simulink model "BMS_CL_Harness_advancedcell"  (R2015b)
settings: Solver=FixedStepDiscrete  StartTime=0.0  StopTime=final_time  FixedStep=BMSk_stepSize  RelTol=1e-3
values from neighbouring files (symbols this model uses):
  charge_cycle = 3    [BMS_test_cases.m]
undefined symbols (not defined in the file or in its folder): BMSc_airTemperature, BMSc_cabinTemperature, BMSk_stepSize, cell_ocvs_sampling, cell_socs_sampling, cell_temps_sampling, cell_voltages_sampling, inital_outlet_temperature, initial_cell_ocvs, initial_cell_socs, initial_cell_temps, initial_cell_voltages, initial_pack_current, initial_pack_soc, initial_pack_voltage, initial_vehicle_side_voltage, pack_current_sampling, pack_soc_sampling, pack_voltage_sampling, sigbuilder_block, vehicle_side_voltage_sampling
libraries: simulink x3
(part 1 of 2)
settings Model: PauseTimes=22  Creator=ms2zwt  LastModifiedBy=nctzv8
settings ConfigSet: Description=OpenECU configuration set for code generation under RTW-EC.
settings SolverCC: PositivePriorityOrder=on
settings DataIOCC: SaveFormat=Array  SignalLoggingSaveFormat=ModelDataLogs  SignalLogging=off
settings OptimizationCC: DefaultParameterBehavior=Inlined  InlineInvariantSignals=on  ExpressionDepthLimit=2147483647  StateBitsets=on  DataBitsets=on  ZeroExternalMemoryAtStartup=off  ZeroInternalMemoryAtStartup=off  NoFixptDivByZeroProtection=on  EfficientFloat2IntCast=on  OptimizeModelRefInitCode=on  LifeSpan=1
settings DebuggingCC: SaveWithParameterizedLinksMsg=none  UnderspecifiedInitializationDetection=Classic  MergeDetectMultiDrivingBlocksExec=none  SignalResolutionControl=TryResolveAllWithWarning  MultiTaskDSMMsg=warning  MultiTaskCondExecSysMsg=none  SingleTaskRateTransMsg=error  CheckMatrixSingularityMsg=warning  VectorMatrixConversionMsg=warning  FcnCallInpInsideContextMsg=UseLocalSettings  SignalLabelMismatchMsg=warning  StateNameClashWarn=warning
settings HardwareCC: ProdBitPerPointer=32  ProdLargestAtomicInteger=Long  ProdLargestAtomicFloat=Double  ProdEndianess=BigEndian  ProdWordSize=32  ProdHWDeviceType=Freescale->32-bit PowerPC  TargetIntDivRoundTo=Zero  TargetEndianess=BigEndian  TargetHWDeviceType=Freescale->32-bit PowerPC  ProdEqTarget=off
settings RTWCC: SystemTargetFile=openecu_ert.tlc  MakeCommand=make_rtw optimized_floating_point=1  TemplateMakefile=openecu_ert_r2015b_64.tmf  Description=OpenECU Platform Target (ERT, optimised floating-point code)  RetainRTWFile=on  IncludeHyperlinkInReport=on
settings CodeAppCC: ForceParamTrailComments=on  IgnoreCustomStorageClasses=off  SimulinkDataObjDesc=on  CustomSymbolStrType=$N$R$M  InsertBlockDesc=on  InternalIdentifier=Classic
settings STFCustomTargetCC: TargetLibSuffix=.a  GenerateSampleERTMain=on  ConcurrentExecutionCompliant=off  IncludeMdlTerminateFcn=off  GeneratePreprocessorConditionals=Use local settings  CombineOutputUpdateFcns=on  IncludeFileDelimiter=UseQuote  ERTCustomFileBanners=on  SupportContinuousTime=off  MATLABClassNameForMDSCustomization=Simulink.SoftwareTarget.ERTCustomization  CPPClassGenCompliant=off  GRTInterface=off  SystemTargetFile=openecu_ert.tlc
settings ERTTargetCC: GenerateSampleERTMain=on  ParMdlRefBuildCompliant=off  CompOptLevelCompliant=off  ConcurrentExecutionCompliant=off  IncludeMdlTerminateFcn=off  ERTFirstTimeCompliant=off  IncludeFileDelimiter=UseQuote  SupportNonInlinedSFcns=on  ModelStepFunctionPrototypeControlCompliant=off  CPPClassGenCompliant=off  UseToolchainInfoCompliant=off  ExtModeMexFile=noextcomm  InlinedParameterPlacement=NonHierarchical  ERTSrcFileBannerTemplate=oe_code_c_template.cgt  ERTHdrFileBannerTemplate=oe_code_h_template.cgt  ERTDataSrcFileTemplate=oe_data_c_template.cgt  ERTDataHdrFileTemplate=oe_data_h_template.cgt  ERTCustomFileTemplate=example_file_process.tlc  GlobalDataDefinition=InSeparateSourceFile  GlobalDataReference=InSeparateHeaderFile  EnableUserReplacementTypes=on

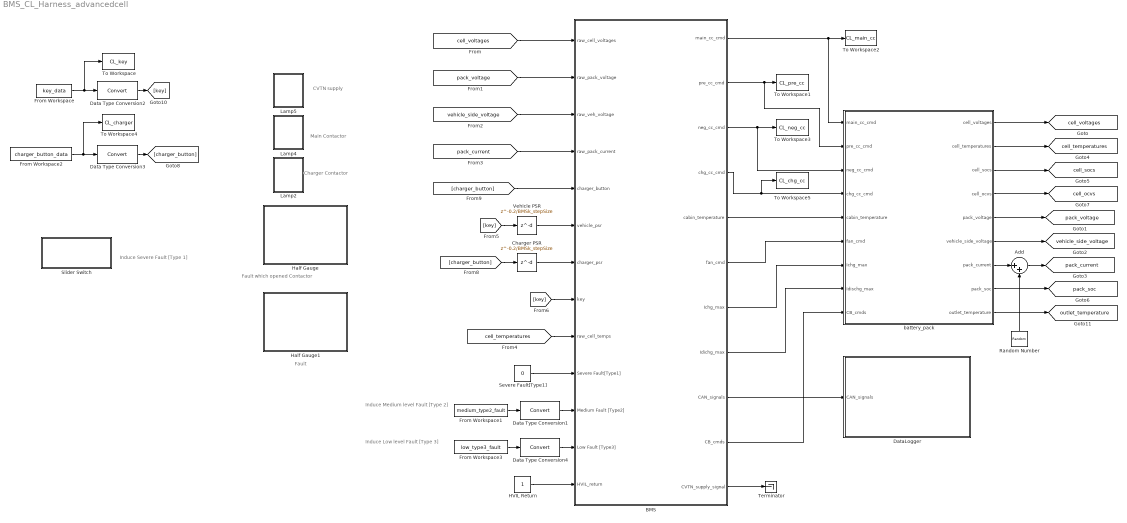
== system BMS_CL_Harness_advancedcell ==
  note: Fault
  note: Induce Medium level Fault
      | [Type 2]
  note: Induce Severe Fault
      | [Type 1]
  note: CVTN supply
  note: Charger Contactor
  note: Main Contactor
  note: Fault which opened Contactor
  note: Induce Low level Fault
      | [Type 3]
  Add : Sum  Inputs=|++
  BMS : Subsystem
  Charger PSR : Delay  DelayLength=0.2/BMSk_stepSize
  Data Type Conversion{1..4} (4 alike) : DataTypeConversion
  DataLogger : Subsystem
  From Workspace : FromWorkspace  VariableName=key_data  SampleTime=BMSk_stepSize
  From Workspace1 : FromWorkspace  VariableName=medium_type2_fault  SampleTime=BMSk_stepSize
  From Workspace2 : FromWorkspace  VariableName=charger_button_data  SampleTime=BMSk_stepSize
  From Workspace3 : FromWorkspace  VariableName=low_type3_fault  SampleTime=BMSk_stepSize
  HVIL Return : Constant  OutDataTypeStr=double  SampleTime=-1
  Half Gauge : Subsystem  DialogController=hmiCreateDDGDialog  IsWebBlock=on  mask(MWDashboardBlock){webBlockId=389, webBlockType=semicirculargauge, ShowInLibBrowser=on, ShowInitialText=on, HMISrcModelName=BMS_CL_Harness_advancedcell}
      mask prompts: webBlockId "WebBlock Id"; webBlockType "WebBlock Type"; HMISrcModelName "Source Model"
      mask Help: helpview([docroot '/mapfiles/simulink.map'], 'hmi_half_gauge')
      mask Display:
      | if strcmp(get_param(bdroot(gcb),'BlockDiagramType'), 'library')
      |     image([(matlabroot) '/toolbox/simulink/hmi/icons/SemicircularGauge.png']);
      | end
  Half Gauge1 : Subsystem  DialogController=hmiCreateDDGDialog  IsWebBlock=on  mask(MWDashboardBlock){webBlockId=61f53593-50c6-4eb0-9ab9-b848c630297d, webBlockType=semicirculargauge, ShowInLibBrowser=on, ShowInitialText=on, HMISrcModelName=BMS_CL_Harness_advancedcell}
      mask prompts: webBlockId "WebBlock Id"; webBlockType "WebBlock Type"; HMISrcModelName "Source Model"
      mask Help: helpview([docroot '/mapfiles/simulink.map'], 'hmi_half_gauge')
      mask Display:
      | if strcmp(get_param(bdroot(gcb),'BlockDiagramType'), 'library')
      |     image([(matlabroot) '/toolbox/simulink/hmi/icons/SemicircularGauge.png']);
      | end
  Lamp2 : Subsystem  DialogController=hmiCreateDDGDialog  IsWebBlock=on  mask(MWDashboardBlock){webBlockId=390, webBlockType=lamp, ShowInLibBrowser=on, ShowInitialText=on, HMISrcModelName=BMS_CL_Harness_advancedcell}
      mask prompts: webBlockType "WebBlock Type"; HMISrcModelName "Source Model"
      mask Help: helpview([docroot '/mapfiles/simulink.map'], 'hmi_lamp')
      mask Display:
      | if strcmp(get_param(bdroot(gcb),'BlockDiagramType'), 'library')
      |     image([(matlabroot) '/toolbox/simulink/hmi/icons/Lamp.png']);
      | end
  Lamp4 : Subsystem  DialogController=hmiCreateDDGDialog  IsWebBlock=on  mask(MWDashboardBlock){webBlockId=392, webBlockType=lamp, ShowInLibBrowser=on, ShowInitialText=on, HMISrcModelName=BMS_CL_Harness_advancedcell}
      mask prompts: webBlockType "WebBlock Type"; HMISrcModelName "Source Model"
      mask Help: helpview([docroot '/mapfiles/simulink.map'], 'hmi_lamp')
      mask Display:
      | if strcmp(get_param(bdroot(gcb),'BlockDiagramType'), 'library')
      |     image([(matlabroot) '/toolbox/simulink/hmi/icons/Lamp.png']);
      | end
  Lamp5 : Subsystem  DialogController=hmiCreateDDGDialog  IsWebBlock=on  mask(MWDashboardBlock){webBlockId=393, webBlockType=lamp, ShowInLibBrowser=on, ShowInitialText=on, HMISrcModelName=BMS_CL_Harness_advancedcell}
      mask prompts: webBlockType "WebBlock Type"; HMISrcModelName "Source Model"
      mask Help: helpview([docroot '/mapfiles/simulink.map'], 'hmi_lamp')
      mask Display:
      | if strcmp(get_param(bdroot(gcb),'BlockDiagramType'), 'library')
      |     image([(matlabroot) '/toolbox/simulink/hmi/icons/Lamp.png']);
      | end
  Random Number : RandomNumber  Variance=0  SampleTime=BMSk_stepSize
  Severe Fault[Type1] : Constant  Value=0  OutDataTypeStr=uint8  SampleTime=-1
  Slider Switch : Subsystem  DialogController=hmiCreateDDGDialog  IsWebBlock=on  mask(MWDashboardBlock){webBlockId=371, webBlockType=sliderswitch, ShowInLibBrowser=on, ShowInitialText=on, HMISrcModelName=BMS_CL_Harness_advancedcell}
      mask prompts: webBlockId "WebBlock Id"; webBlockType "WebBlock Type"; HMISrcModelName "Source Model"
      mask Help: helpview([docroot '/mapfiles/simulink.map'], 'hmi_slider_switch')
      mask Display:
      | if strcmp(get_param(bdroot(gcb),'BlockDiagramType'), 'library')
      |     image([(matlabroot) '/toolbox/simulink/hmi/icons/SliderSwitch.png']);
      | end
  Terminator : Terminator
  To Workspace : ToWorkspace  VariableName=CL_key  SaveFormat=Timeseries  SampleTime=-1
  To Workspace1 : ToWorkspace  VariableName=CL_pre_cc  SaveFormat=Timeseries  SampleTime=-1
  To Workspace2 : ToWorkspace  VariableName=CL_main_cc  SaveFormat=Timeseries  SampleTime=-1
  To Workspace3 : ToWorkspace  VariableName=CL_neg_cc  SaveFormat=Timeseries  SampleTime=-1
  To Workspace4 : ToWorkspace  VariableName=CL_charger  SaveFormat=Timeseries  SampleTime=-1
  To Workspace5 : ToWorkspace  VariableName=CL_chg_cc  SaveFormat=Timeseries  SampleTime=-1
  Vehicle PSR : Delay  DelayLength=0.2/BMSk_stepSize
  battery_pack : Subsystem
  tag scope: cell_ocvs=global, cell_socs=global, cell_temperatures=global, cell_voltages=global, outlet_temperature=global, pack_current=global, pack_soc=global, pack_voltage=global, vehicle_side_voltage=global
  wires:
  battery_pack/1(cell_voltages) -> [cell_voltages]
  battery_pack/2(cell_temperatures) -> [cell_temperatures]
  battery_pack/3(cell_socs) -> [cell_socs]
  battery_pack/4(cell_ocvs) -> [cell_ocvs]
  battery_pack/5(pack_voltage) -> [pack_voltage]
  battery_pack/6(vehicle_side_voltage) -> [vehicle_side_voltage]
  battery_pack/8(pack_soc) -> [pack_soc]
  [cell_temperatures] -> BMS/9(raw_cell_temps)
  Vehicle PSR/1 -> BMS/6(vehicle_psr)
  [key] -> Vehicle PSR/1
  [key] -> BMS/8(key)
  [charger_button] -> BMS/5(charger_button)
  Add/1 -> [pack_current]
  battery_pack/7(pack_current) -> Add/1
  Random Number/1 -> Add/2
  Charger PSR/1 -> BMS/7(charger_psr)
  [charger_button] -> Charger PSR/1
  BMS/4(chg_cc_cmd) -> To Workspace5/1, battery_pack/4(chg_cc_cmd)
  BMS/3(neg_cc_cmd) -> battery_pack/3(neg_cc_cmd), To Workspace3/1
  BMS/1(main_cc_cmd) -> battery_pack/1(main_cc_cmd), To Workspace2/1
  BMS/5(cabin_temperature) -> battery_pack/5(cabin_temperature)
  BMS/6(fan_cmd) -> battery_pack/6(fan_cmd)
  battery_pack/9(outlet_temperature) -> [outlet_temperature]
  Data Type Conversion2/1 -> [key]
  Data Type Conversion4/1 -> BMS/12(Low Fault [Type3])
  From Workspace1/1 -> Data Type Conversion1/1
  Severe Fault[Type1]/1 -> BMS/10(Severe Fault[Type1])
  [pack_current] -> BMS/4(raw_pack_current)
  [vehicle_side_voltage] -> BMS/3(raw_veh_voltage)
  [pack_voltage] -> BMS/2(raw_pack_voltage)
  [cell_voltages] -> BMS/1(raw_cell_voltages)
  BMS/9(CAN_signals) -> DataLogger/1(CAN_signals)
  BMS/10(CB_cmds) -> battery_pack/9(CB_cmds)
  BMS/2(pre_cc_cmd) -> battery_pack/2(pre_cc_cmd), To Workspace1/1
  BMS/7(Ichg_max) -> battery_pack/7(Ichg_max)
  BMS/8(Idichg_max) -> battery_pack/8(Idischg_max)
  Data Type Conversion3/1 -> [charger_button]
  From Workspace/1 -> To Workspace/1, Data Type Conversion2/1
  From Workspace2/1 -> To Workspace4/1, Data Type Conversion3/1
  Data Type Conversion1/1 -> BMS/11(Medium Fault [Type2])
  BMS/11(CVTN_supply_signal) -> Terminator/1
  HVIL Return/1 -> BMS/13(HVIL_return)
  From Workspace3/1 -> Data Type Conversion4/1

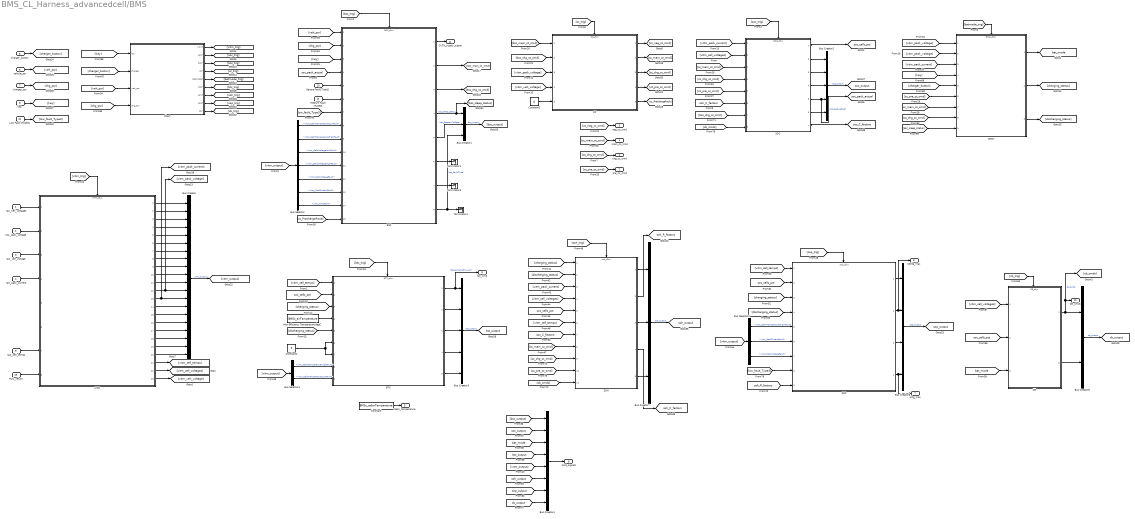
== system BMS_CL_Harness_advancedcell/BMS ==
  raw_cell_voltages : Inport
  raw_pack_voltage : Inport  Port=2
  raw_veh_voltage : Inport  Port=3
  raw_pack_current : Inport  Port=4
  charger_button : Inport  Port=5  OutDataTypeStr=uint8
  vehicle_psr : Inport  Port=6
  charger_psr : Inport  Port=7
  key : Inport  Port=8  OutDataTypeStr=uint8
  raw_cell_temps : Inport  Port=9
  Severe Fault[Type1] : Inport  Port=10
  Medium Fault [Type2] : Inport  Port=11
  Low Fault [Type3] : Inport  Port=12
  HVIL_return : Inport  Port=13  OutDataTypeStr=double
  BMO : ModelReference  ModelNameDialog=BMO_sfun.slx  SimulationMode=Normal  Variant=on  ModelReferenceVersion=1.4  CopyOfModelName=BMO_sfun.slx  TriggerPortName=Trigger  TriggerPortTriggerType=function-call  TriggerPortStatesWhenEnabling=held
  BSC : ModelReference  ModelNameDialog=BSC_sfun.slx  SimulationMode=Normal  Variant=on  ModelReferenceVersion=1.2  CopyOfModelName=BSC_sfun.slx  TriggerPortName=Trigger  TriggerPortTriggerType=function-call  TriggerPortStatesWhenEnabling=held
  BTC : ModelReference  ModelNameDialog=BTC_sfun.slx  SimulationMode=Normal  Variant=on  ModelReferenceVersion=1.3  CopyOfModelName=BTC_sfun.slx  TriggerPortName=Trigger  TriggerPortTriggerType=function-call  TriggerPortStatesWhenEnabling=held
  Bus Creator : BusCreator  Inputs=20
  Bus Creator1 : BusCreator  Inputs=3
  Bus Creator2 : BusCreator  Inputs=5
  Bus Creator3 : BusCreator  Inputs=5
  Bus Creator4 : BusCreator  Inputs=8
  Bus Creator5 : BusCreator  Inputs=4
  Bus Creator6 : BusCreator  Inputs=2
  Bus Creator7 : BusCreator  Inputs=3
  Bus Selector : BusSelector  OutputSignals=vitm_CellsTemperatureLowFault,vitm_CellsTemperatureHighFault,vitm_CellsVoltageLowFault,vitm_CellsVoltageHighFault,vitm_PackVoltageFault,vitm_PackCurrentFault,vitm_HVILFault
  Bus Selector1 : BusSelector  OutputSignals=vitm_CellsTemperatureHighFault,vitm_CellsTemperatureLowFault
  Bus Selector2 : BusSelector  OutputSignals=vitm_CellsTemperatureHighFault,vitm_PackCurrentFault,vitm_PackVoltageFault
  CB : ModelReference  ModelNameDialog=CB_sfun.slx  SimulationMode=Normal  Variant=on  ModelReferenceVersion=1.3  CopyOfModelName=CB_sfun.slx  TriggerPortName=Trigger  TriggerPortTriggerType=function-call  TriggerPortStatesWhenEnabling=held
  CC : ModelReference  ModelNameDialog=CC_sfun.slx  SimulationMode=Normal  Variant=on  ModelReferenceVersion=1.2  CopyOfModelName=CC_sfun.slx  TriggerPortName=Trigger  TriggerPortTriggerType=function-call  TriggerPortStatesWhenEnabling=held
  Chart : Stateflow chart  TreatAsAtomicUnit=on
  Constant : Constant  Value=BMSc_cabinTemperature  SampleTime=BMSk_stepSize
  Constant1 : Constant  Value=0  OutDataTypeStr=boolean  SampleTime=-1
  Constant2 : Constant  Value=0  OutDataTypeStr=double  SampleTime=-1
  Max Efficiency Temperature degC : Constant  Value=BMSc_airTemperature  SampleTime=BMSk_stepSize
  SOC : ModelReference  ModelNameDialog=SOC_sfun.slx  SimulationMode=Normal  Variant=on  ModelReferenceVersion=1.25  CopyOfModelName=SOC_sfun.slx  TriggerPortName=Trigger  TriggerPortTriggerType=function-call  TriggerPortStatesWhenEnabling=held
  SOH : ModelReference  ModelNameDialog=soh_sfun.slx  SimulationMode=Normal  Variant=on  ModelReferenceVersion=1.3  CopyOfModelName=soh_sfun.slx  TriggerPortName=Trigger  TriggerPortTriggerType=function-call  TriggerPortStatesWhenEnabling=held
  SOP : ModelReference  ModelNameDialog=sop_sfun.slx  SimulationMode=Normal  Variant=on  ModelReferenceVersion=1.4  CopyOfModelName=sop_sfun.slx  TriggerPortName=Trigger  TriggerPortTriggerType=function-call  TriggerPortStatesWhenEnabling=held
  Terminator1 : Terminator
  Terminator3 : Terminator
  Terminator4 : Terminator
  VITM : ModelReference  ModelNameDialog=VITM_sfun.slx  SimulationMode=Normal  Variant=on  ModelReferenceVersion=1.3  CopyOfModelName=VITM_sfun.slx  TriggerPortName=Trigger  TriggerPortTriggerType=function-call  TriggerPortStatesWhenEnabling=held
  main_cc_cmd : Outport
  pre_cc_cmd : Outport  Port=2
  neg_cc_cmd : Outport  Port=3
  chg_cc_cmd : Outport  Port=4
  cabin_temperature : Outport  Port=5
  fan_cmd : Outport  Port=6
  Ichg_max : Outport  Port=7
  Idichg_max : Outport  Port=8
  CAN_signals : Outport  Port=9
  CB_cmds : Outport  Port=10
  CVTN_supply_signal : Outport  Port=11
  tag scope: bat_mode=global, btc_output=global, cb_output=global, soc_C_factors=global, soc_cells_pct=global, soc_output=global, soc_pack_actual=global, soh_C_factors=global, soh_R_factors=global, soh_output=global, sop_output=global
  wires:
  SOC/1 -> [soc_cells_pct]
  [vitm_pack_voltage] -> BMO/1
  BMO/1 -> [bat_mode]
  [vitm_cell_voltages] -> SOC/2
  Chart/1(vitm()) -> [vitm_trig]
  Chart/2(soc()) -> [soc_trig]
  Chart/3(bsc()) -> [bsc_trig]
  Chart/4(cc()) -> [cc_trig]
  Chart/5(batmode()) -> [batmode_trig]
  [soc_trig] -> SOC/Trigger
  [batmode_trig] -> BMO/Trigger
  [cc_trig] -> CC/Trigger
  Constant/1 -> cabin_temperature/1
  Max Efficiency Temperature degC/1 -> BTC/4
  [vitm_cell_temps] -> BTC/1
  [soc_cells_pct] -> BTC/2
  BMO/2 -> [charging_status]
  BMO/3 -> [discharging_status]
  [charging_status] -> BTC/3
  [discharging_status] -> BTC/5
  Constant1/1 -> BTC/6, BTC/7
  raw_cell_voltages/1 -> VITM/1
  [vitm_pack_current] -> SOC/1
  [vitm_pack_current] -> BMO/3
  [vitm_pack_voltage] -> BMO/2
  [bsc_main_cc_cmd] -> CC/1
  [bsc_chg_cc_cmd] -> CC/2
  CC/1 -> [cc_neg_cc_cmd]
  CC/2 -> [cc_main_cc_cmd]
  CC/3 -> [cc_chg_cc_cmd]
  CC/4 -> [cc_pre_cc_cmd]
  [cc_neg_cc_cmd] -> neg_cc_cmd/1
  [cc_main_cc_cmd] -> main_cc_cmd/1
  [cc_chg_cc_cmd] -> chg_cc_cmd/1
  [cc_pre_cc_cmd] -> pre_cc_cmd/1
  [cc_main_cc_cmd] -> SOC/3
  Chart/6(btc()) -> [btc_trig]
  VITM/1 -> Bus Creator/1
  VITM/2 -> Bus Creator/2
  VITM/3 -> Bus Creator/3
  VITM/4 -> Bus Creator/4
  VITM/5 -> Bus Creator/5
  VITM/6 -> Bus Creator/6
  VITM/7 -> Bus Creator/7
  VITM/8 -> Bus Creator/8
  VITM/9 -> Bus Creator/9
  VITM/10 -> Bus Creator/10
  VITM/11 -> Bus Creator/11
  VITM/12 -> [vitm_pack_voltage], Bus Creator/12
  VITM/13 -> [vitm_pack_current], Bus Creator/13
  VITM/14 -> Bus Creator/14
  VITM/15 -> Bus Creator/15
  VITM/16 -> Bus Creator/16
  VITM/17 -> Bus Creator/17
  VITM/18 -> Bus Creator/18
  VITM/19 -> Bus Creator/19
  Bus Creator/1 -> [vitm_output]  "vitm_output"
  [vitm_output] -> Bus Selector/1
  [btc_trig] -> BTC/Trigger
  raw_pack_voltage/1 -> VITM/2
  raw_pack_current/1 -> VITM/4
  raw_cell_temps/1 -> VITM/7
  CC/5 -> [cc_PrechargeFault]
  raw_veh_voltage/1 -> VITM/3
  charger_button/1 -> [charger_button]
  vehicle_psr/1 -> [veh_psr]
  [veh_psr] -> Chart/3(veh_psr)
  [vitm_output] -> Bus Selector1/1
  Bus Selector1/1 -> BTC/8  "<vitm_CellsTemperatureHighFault>"
  Bus Selector1/2 -> BTC/9  "<vitm_CellsTemperatureLowFault>"
  Bus Creator1/1 -> [bsc_output]  "bsc_output"
  SOC/2 -> Bus Creator2/1
  SOC/3 -> Bus Creator2/2
  SOC/4 -> Bus Creator2/3
  SOC/5 -> Bus Creator2/4, [soc_pack_actual]  "soc_pack_actual"
  SOC/6 -> Bus Creator2/5
  Bus Creator2/1 -> [soc_output]  "soc_output"
  BTC/1 -> fan_cmd/1, Bus Creator3/1  "btc_coolant_flow_pct"
  BTC/2 -> Bus Creator3/2
  BTC/3 -> Bus Creator3/3
  BTC/4 -> Bus Creator3/4
  BTC/5 -> Bus Creator3/5
  Bus Creator3/1 -> [btc_output]  "btc_output"
  [bsc_output] -> Bus Creator4/1
  [soc_output] -> Bus Creator4/2
  [bat_mode] -> Bus Creator4/3
  [btc_output] -> Bus Creator4/4
  [vitm_output] -> Bus Creator4/5
  Bus Creator4/1 -> CAN_signals/1
  [charging_status] -> SOH/1
  [discharging_status] -> SOH/2
  [vitm_pack_current] -> SOH/3
  [vitm_cell_voltages] -> SOH/4
  [soc_cells_pct] -> SOH/5
  [vitm_cell_temps] -> SOH/6
  Chart/7(soh()) -> [soh_trig]
  Chart/8(sop()) -> [sop_trig]
  [vitm_cell_temps] -> SOP/1
  [soc_cells_pct] -> SOP/2
  [charging_status] -> SOP/3
  [discharging_status] -> SOP/4
  [vitm_output] -> Bus Selector2/1
  Bus Selector2/1 -> SOP/5  "<vitm_CellsTemperatureHighFault>"
  Bus Selector2/2 -> SOP/6  "<vitm_PackCurrentFault>"
  Bus Selector2/3 -> SOP/7  "<vitm_PackVoltageFault>"
  Chart/9(cb()) -> [cb_trig]
  [cb_trig] -> CB/Trigger
  [soc_cells_pct] -> CB/2
  [vitm_cell_voltages] -> CB/1
  [bat_mode] -> CB/3
  SOP/1 -> Bus Creator5/1
  SOP/2 -> Bus Creator5/2, Idichg_max/1
  SOP/3 -> Bus Creator5/3
  SOP/4 -> Ichg_max/1, Bus Creator5/4
  Bus Creator5/1 -> [sop_output]  "sop_output"
  [cc_pre_cc_cmd] -> SOC/5
  [cc_chg_cc_cmd] -> SOC/4
  [sop_output] -> Bus Creator4/7
  CB/2 -> Bus Creator6/2
  charger_psr/1 -> [chg_psr]
  [chg_psr] -> Chart/4(chg_psr)
  key/1 -> [key]
  [charger_button] -> Chart/2(charger)
  [key] -> Chart/1(key)
  [cc_pre_cc_cmd] -> BMO/6
  [cc_main_cc_cmd] -> BMO/7
  [cc_chg_cc_cmd] -> BMO/8
  [bsc_sleep_status] -> BMO/9
  [key] -> BMO/4
  [charger_button] -> BMO/5
  [vitm_pack_voltage] -> CC/3
  [vitm_veh_voltage] -> CC/4
  Constant2/1 -> CC/5
  SOC/7 -> [soc_C_factors]
  [soc_C_factors] -> SOH/7
  [soh_C_factors] -> SOC/6
  [bsc_chg_cc_cmd] -> SOC/7
  CB/1 -> Bus Creator6/1, [cb_cmds], CB_cmds/1  "cb_cmds"
  [cc_main_cc_cmd] -> SOH/8
  [cc_pre_cc_cmd] -> SOH/10
  [cc_chg_cc_cmd] -> SOH/9
  [cb_cmds] -> SOC/8
  [cb_cmds] -> SOH/11
  Bus Creator6/1 -> [cb_output]  "cb_output"
  [cb_output] -> Bus Creator4/8
  SOH/1 -> Bus Creator7/1
  SOH/3 -> Bus Creator7/2
  SOH/5 -> Bus Creator7/3
  SOH/2 -> [soh_R_factors]
  SOH/4 -> [soh_C_factors]
  Bus Creator7/1 -> [soh_output]  "soh_output"
  [soh_output] -> Bus Creator4/6
  HVIL_return/1 -> VITM/8
  VITM/20 -> Bus Creator/20
  VITM/21 -> [vitm_cell_temps]
  VITM/22 -> [vitm_cell_voltages]
  VITM/23 -> [vitm_veh_voltage]
  [soh_R_factors] -> SOP/9
  Low Fault [Type3]/1 -> [low_fault_Type3]
  [low_fault_Type3] -> SOP/8
  BSC/4 -> [bsc_sleep_status], Bus Creator1/1  "bsc_sleep_status"
  [veh_psr] -> BSC/1
  [chg_psr] -> BSC/2
  [key] -> BSC/3
  [soc_pack_actual] -> BSC/4
  Severe Fault[Type1]/1 -> BSC/5
  Medium Fault [Type2]/1 -> BSC/6
  [low_fault_Type3] -> BSC/7
  Bus Selector/1 -> BSC/8  "<vitm_CellsTemperatureLowFault>"
  Bus Selector/2 -> BSC/9  "<vitm_CellsTemperatureHighFault>"
  Bus Selector/3 -> BSC/10  "<vitm_CellsVoltageLowFault>"
  Bus Selector/4 -> BSC/11  "<vitm_CellsVoltageHighFault>"
  Bus Selector/5 -> BSC/12  "<vitm_PackVoltageFault>"
  Bus Selector/6 -> BSC/13  "<vitm_PackCurrentFault>"
  Bus Selector/7 -> BSC/14  "<vitm_HVILFault>"
  [cc_PrechargeFault] -> BSC/15
  BSC/1 -> CVTN_supply_signal/1
  BSC/2 -> [bsc_main_cc_cmd]
  BSC/3 -> [bsc_chg_cc_cmd]
  BSC/5 -> Bus Creator1/2  "bsc_ReasonToOpen"
  BSC/7 -> Terminator3/1
  BSC/8 -> Bus Creator1/3, Terminator4/1  "bsc_FaultType"
  [bsc_trig] -> BSC/Trigger
  BSC/6 -> Terminator1/1
  [soh_trig] -> SOH/Trigger
  [sop_trig] -> SOP/Trigger
  [vitm_trig] -> VITM/Trigger

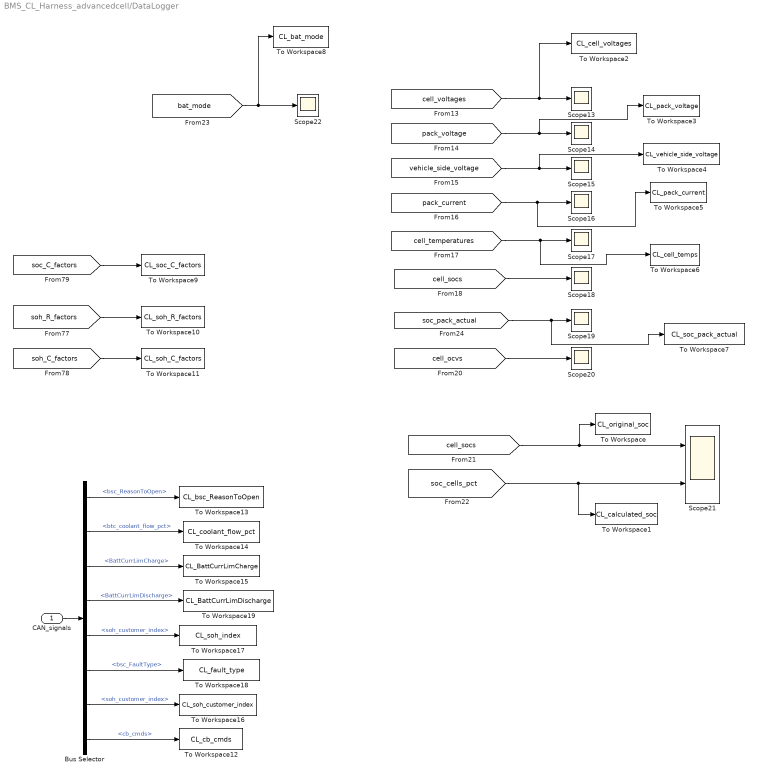
== system BMS_CL_Harness_advancedcell/DataLogger ==
  CAN_signals : Inport
  Bus Selector : BusSelector  OutputSignals=bsc_output.bsc_ReasonToOpen,btc_output.btc_coolant_flow_pct,sop_output.BattCurrLimCharge,sop_output.BattCurrLimDischarge,soh_output.soh_customer_index,bsc_output.bsc_FaultType,soh_output.soh_customer_index,cb_output.cb_cmds
  Scope{13..20,22} (9 alike) : Scope
  Scope21 : Scope  NumInputPorts=2
  To Workspace : ToWorkspace  VariableName=CL_original_soc  SaveFormat=Timeseries  SampleTime=-1
  To Workspace1 : ToWorkspace  VariableName=CL_calculated_soc  SaveFormat=Timeseries  SampleTime=-1
  To Workspace10 : ToWorkspace  VariableName=CL_soh_R_factors  SaveFormat=Timeseries  SampleTime=-1
  To Workspace11 : ToWorkspace  VariableName=CL_soh_C_factors  SaveFormat=Timeseries  SampleTime=-1
  To Workspace12 : ToWorkspace  VariableName=CL_cb_cmds  SaveFormat=Timeseries  SampleTime=-1
  To Workspace13 : ToWorkspace  VariableName=CL_bsc_ReasonToOpen  SaveFormat=Timeseries  SampleTime=-1
  To Workspace14 : ToWorkspace  VariableName=CL_coolant_flow_pct  SaveFormat=Timeseries  SampleTime=-1
  To Workspace15 : ToWorkspace  VariableName=CL_BattCurrLimCharge  SaveFormat=Timeseries  SampleTime=-1
  To Workspace16 : ToWorkspace  VariableName=CL_soh_customer_index  SaveFormat=Timeseries  SampleTime=-1
  To Workspace17 : ToWorkspace  VariableName=CL_soh_index  SaveFormat=Timeseries  SampleTime=-1
  To Workspace18 : ToWorkspace  VariableName=CL_fault_type  SaveFormat=Timeseries  SampleTime=-1
  To Workspace19 : ToWorkspace  VariableName=CL_BattCurrLimDischarge  SaveFormat=Timeseries  SampleTime=-1
  To Workspace2 : ToWorkspace  VariableName=CL_cell_voltages  SaveFormat=Timeseries  SampleTime=-1
  To Workspace3 : ToWorkspace  VariableName=CL_pack_voltage  SaveFormat=Timeseries  SampleTime=-1
  To Workspace4 : ToWorkspace  VariableName=CL_vehicle_side_voltage  SaveFormat=Timeseries  SampleTime=-1
  To Workspace5 : ToWorkspace  VariableName=CL_pack_current  SaveFormat=Timeseries  SampleTime=-1
  To Workspace6 : ToWorkspace  VariableName=CL_cell_temps  SaveFormat=Timeseries  SampleTime=-1
  To Workspace7 : ToWorkspace  VariableName=CL_soc_pack_actual  SaveFormat=Timeseries  SampleTime=-1
  To Workspace8 : ToWorkspace  VariableName=CL_bat_mode  SaveFormat=Timeseries  SampleTime=-1
  To Workspace9 : ToWorkspace  VariableName=CL_soc_C_factors  SaveFormat=Timeseries  SampleTime=-1
  wires:
  [cell_voltages] -> To Workspace2/1, Scope13/1
  [pack_voltage] -> To Workspace3/1, Scope14/1
  [vehicle_side_voltage] -> To Workspace4/1, Scope15/1
  [pack_current] -> To Workspace5/1, Scope16/1
  [cell_temperatures] -> To Workspace6/1, Scope17/1
  [cell_socs] -> Scope18/1
  [cell_ocvs] -> Scope20/1
  [cell_socs] -> To Workspace/1, Scope21/1
  [bat_mode] -> To Workspace8/1, Scope22/1
  [soc_cells_pct] -> To Workspace1/1, Scope21/2
  [soc_pack_actual] -> To Workspace7/1, Scope19/1
  [soc_C_factors] -> To Workspace9/1
  [soh_C_factors] -> To Workspace11/1
  [soh_R_factors] -> To Workspace10/1
  CAN_signals/1 -> Bus Selector/1
  Bus Selector/1 -> To Workspace13/1  "<bsc_ReasonToOpen>"
  Bus Selector/2 -> To Workspace14/1  "<btc_coolant_flow_pct>"
  Bus Selector/3 -> To Workspace15/1  "<BattCurrLimCharge>"
  Bus Selector/7 -> To Workspace16/1  "<soh_customer_index>"
  Bus Selector/6 -> To Workspace18/1  "<bsc_FaultType>"
  Bus Selector/5 -> To Workspace17/1  "<soh_customer_index>"
  Bus Selector/4 -> To Workspace19/1  "<BattCurrLimDischarge>"
  Bus Selector/8 -> To Workspace12/1  "<cb_cmds>"

== system BMS_CL_Harness_advancedcell/Half Gauge ==

== system BMS_CL_Harness_advancedcell/Half Gauge1 ==

== system BMS_CL_Harness_advancedcell/Lamp2 ==

== system BMS_CL_Harness_advancedcell/Lamp4 ==

== system BMS_CL_Harness_advancedcell/Lamp5 ==

== system BMS_CL_Harness_advancedcell/Slider Switch ==

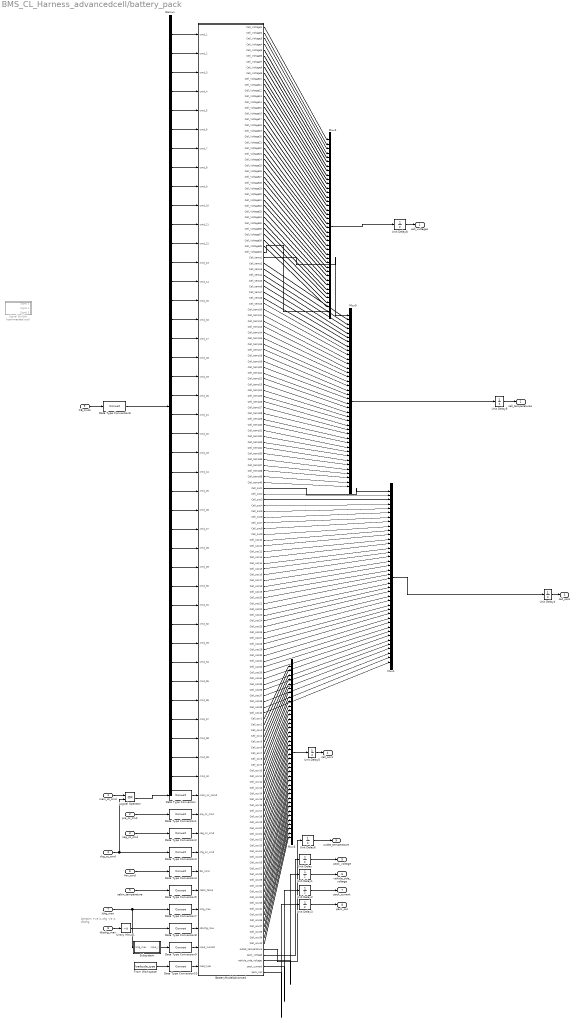
== system BMS_CL_Harness_advancedcell/battery_pack ==
  note: Amesim
      | +ve is chg
      | -ve is dischg
  main_cc_cmd : Inport
  pre_cc_cmd : Inport  Port=2
  neg_cc_cmd : Inport  Port=3
  chg_cc_cmd : Inport  Port=4
  cabin_temperature : Inport  Port=5
  fan_cmd : Inport  Port=6
  Ichg_max : Inport  Port=7
  Idischg_max : Inport  Port=8
  CB_cmds : Inport  Port=9
  BatteryModelAdvanced : Subsystem  Tag=AME2SLCoSim  InitFcn=AMESimLib_initBlock  StartFcn=AMESimLib_startBlock  StopFcn=AMESimLib_stopBlock
      settings: DeleteFcn=AMESimLib_deleteBlock  OpenFcn=AMESimLib_openBlock('AME2SLCoSim')
      mask Display: image(imread('amesim_pix256.png'),[0.4,0.7,0.2,0.2]);disp('Simcenter Amesim co-Sim:\nBatteryModelAdvanced');port_label('input',1,'cmd_1');port_label('input',2,'cmd_2');port_label('input',3,'cmd_3');port_label('input',4,'cmd_4');port_label('input',5,'cmd_5');port_label('input',6,'cmd_6');port_label('input',7,'cmd_7');port_label('input',8,'cmd_8');port_label('input',9,'cmd_9');port_label('input',10,'cmd_10');port_label('input',11,'cmd_11');port_label('input',12,'cmd_12');port_label('input',13,'cmd_13');port_label('input',14,'cmd_14');port_label('input',15,'cmd_15');port_label('input',16,'cmd_16');port_label('input',17,'cmd_17');port_label('input',18,'cmd_18');port_label('input',19,'cmd_19');port_label('input',20,'cmd_20');port_label('input',21,'cmd_21');port_label('input',22,'cmd_22');port_label('input',23,'cmd_23');port_label('input',24,'cmd_24');port_label('input',25,'cmd_25');port_label('input',26,'cmd_26');port_label('input',27,'cmd_27');port_label('input',28,'cmd_28');port_label('input',29,'cmd_29');port_label('input',30,'cmd_30');port_label('input',31,'cmd_31');port_label('input',32,'cmd_32');port_label('input',33,'cmd_33');port_label('input',34,'cmd_34');port_label('input',35,'cmd_35');port_label('input',36,'cmd_36');port_label('input',37,'cmd_37');port_label('input',38,'cmd_38');port_label('input',39,'cmd_39');port_label('input',40,'cmd_40');port_label('input',41,'main_cc_comd');port_label('input',42,'pre_cc_cmd');port_label('input',43,'neg_cc_cmd');port_label('input',44,'chg_cc_cmd');port_label('input',45,'fan_cmd');port_label('input',46,'cabin_temp');port_label('input',47,'Ichg_max');port_label('input',48,'Idischg_max');port_label('input',49,'input_current');port_label('input',50,'load_type');port_label('output',1,'Cell_Voltage1');port_label('output',2,'Cell_Voltage2');port_label('output',3,'Cell_Voltage3');port_label('output',4,'Cell_Voltage4');port_label('output',5,'Cell_Voltage5');port_label('output',6,'Cell_Voltage6');port_label('output',7,'Cell_Voltage7');port_label('output',8,'Cell_Voltage8');port_label('output',9,'Cell_Voltage9');port_label('output',10,'Cell_Voltage10');port_label('output',11,'Cell_Voltage11');port_label('output',12,'Cell_Voltage12');port_label('output',13,'Cell_Voltage13');port_label('output',14,'Cell_Voltage14');port_label('output',15,'Cell_Voltage15');port_label('output',16,'Cell_Voltage16');port_label('output',17,'Cell_Voltage17');port_label('output',18,'Cell_Voltage18');port_label('output',19,'Cell_Voltage19');port_label('output',20,'Cell_Voltage20');port_label('output',21,'Cell_Voltage21');port_label('output',22,'Cell_Voltage22');port_label('output',23,'Cell_Voltage23');port_label('output',24,'Cell_Voltage24');port_label('output',25,'Cell_Voltage25');port_label('output',26,'Cell_Voltage26');port_label('output',27,'Cell_Voltage27');port_label('output',28,'Cell_Voltage28');port_label('output',29,'Cell_Voltage29');port_label('output',30,'Cell_Voltage30');port_label('output',31,'Cell_Voltage31');port_label('output',32,'Cell_Voltage32');port_label('output',33,'Cell_Voltage33');port_label('output',34,'Cell_Voltage34');port_label('output',35,'Cell_Voltage35');port_label('output',36,'Cell_Voltage36');port_label('output',37,'Cell_Voltage37');port_label('output',38,'Cell_Voltage38');port_label('output',39,'Cell_Voltage39');port_label('output',40,'Cell_Voltage40');port_label('output',41,'Cell_temp1');port_label('output',42,'Cell_temp2');port_label('output',43,'Cell_temp3');port_label('output',44,'Cell_temp4');port_label('output',45,'Cell_temp5');port_label('output',46,'Cell_temp6');port_label('output',47,'Cell_temp7');port_label('output',48,'Cell_temp8');port_label('output',49,'Cell_temp9');port_label('output',50,'Cell_temp10');port_label('output',51,'Cell_temp11');port_label('output',52,'Cell_temp12');port_label('output',53,'Cell_temp13');port_label('output',54,'Cell_temp14');port_label('output',55,'Cell_temp15');port_label('output',56,'Cell_temp16');port_label('output',57,'Cell_temp17');port_label('output',58,'Cell_temp18');port_label('output',59,'Cell_temp19');port_label('output',60,'Cell_temp20');port_label('output',61,'Cell_temp21');port_label('output',62,'Cell_temp22');port_label('output',63,'Cell_temp23');port_label('output',64,'Cell_temp24');port_label('output',65,'Cell_temp25');port_label('output',66,'Cell_temp26');port_label('output',67,'Cell_temp27');port_label('output',68,'Cell_temp28');port_label('output',69,'Cell_temp29');port_label('output',70,'Cell_temp30');port_label('output',71,'Cell_temp31');port_label('output',72,'Cell_temp32');port_label('output',73,'Cell_temp33');port_label('output',74,'Cell_temp34');port_label('output',75,'Cell_temp35');port_label('output',76,'Cell_temp36');port_label('output',77,'Cell_temp37');port_label('output',78,'Cell_temp38');port_label('output',79,'Cell_temp39');port_label('output',80,'Cell_temp40');port_label('output',81,'Cell_soc1');port_label('output',82,'Cell_soc2');port_label('output',83,'Cell_soc3');port_label('output',84,'Cell_soc4');port_label('output',85,'Cell_soc5');port_label('output',86,'Cell_soc6');port_label('output',87,'Cell_soc7');port_label('output',88,'Cell_soc8');port_label('output',89,'Cell_soc9');port_label('output',90,'Cell_soc10');port_label('output',91,'Cell_soc11');port_label('output',92,'Cell_soc12');port_label('output',93,'Cell_soc13');port_label('output',94,'Cell_soc14');port_label('output',95,'Cell_soc15');port_label('output',96,'Cell_soc16');port_label('output',97,'Cell_soc17');port_label('output',98,'Cell_soc18');port_label('output',99,'Cell_soc19');port_label('output',100,'Cell_soc20');port_label('output',101,'Cell_soc21');port_label('output',102,'Cell_soc22');port_label('output',103,'Cell_soc23');port_label('output',104,'Cell_soc24');port_label('output',105,'Cell_soc25');port_label('output',106,'Cell_soc26');port_label('output',107,'Cell_soc27');port_label('output',108,'Cell_soc28');port_label('output',109,'Cell_soc29');port_label('output',110,'Cell_soc30');port_label('output',111,'Cell_soc31');port_label('output',112,'Cell_soc32');port_label('output',113,'Cell_soc33');port_label('output',114,'Cell_soc34');port_label('output',115,'Cell_soc35');port_label('output',116,'Cell_soc36');port_label('output',117,'Cell_soc37');port_label('output',118,'Cell_soc38');port_label('output',119,'Cell_soc39');port_label('output',120,'Cell_soc40');port_label('output',121,'Cell_ocv1');port_label('output',122,'Cell_ocv2');port_label('output',123,'Cell_ocv3');port_label('output',124,'Cell_ocv4');port_label('output',125,'Cell_ocv5');port_label('output',126,'Cell_ocv6');port_label('output',127,'Cell_ocv7');port_label('output',128,'Cell_ocv8');port_label('output',129,'Cell_ocv9');port_label('output',130,'Cell_ocv10');port_label('output',131,'Cell_ocv11');port_label('output',132,'Cell_ocv12');port_label('output',133,'Cell_ocv13');port_label('output',134,'Cell_ocv14');port_label('output',135,'Cell_ocv15');port_label('output',136,'Cell_ocv16');port_label('output',137,'Cell_ocv17');port_label('output',138,'Cell_ocv18');port_label('output',139,'Cell_ocv19');port_label('output',140,'Cell_ocv20');port_label('output',141,'Cell_ocv21');port_label('output',142,'Cell_ocv22');port_label('output',143,'Cell_ocv23');port_label('output',144,'Cell_ocv24');port_label('output',145,'Cell_ocv25');port_label('output',146,'Cell_ocv26');port_label('output',147,'Cell_ocv27');port_label('output',148,'Cell_ocv28');port_label('output',149,'Cell_ocv29');port_label('output',150,'Cell_ocv30');port_label('output',151,'Cell_ocv31');port_label('output',152,'Cell_ocv32');port_label('output',153,'Cell_ocv33');port_label('output',154,'Cell_ocv34');port_label('output',155,'Cell_ocv35');port_label('output',156,'Cell_ocv36');port_label('output',157,'Cell_ocv37');port_label('output',158,'Cell_ocv38');port_label('output',159,'Cell_ocv39');port_label('output',160,'Cell_ocv40');port_label('output',161,'outlet_temperature');port_label('output',162,'pack_voltage');port_label('output',163,'vehicle_side_voltage');port_label('output',164,'pack_current');port_label('output',165,'pack_soc');
  Data Type Conversion{,1..10} (11 alike) : DataTypeConversion
  Demux : Demux  Outputs=40
  From Workspace : FromWorkspace  VariableName=loadcycle_type
  Logical Operator : Logic  Operator=OR  AllPortsSameDT=off  OutDataTypeStr=boolean
  Mux{1,4..6} (4 alike) : Mux  Inputs=40
  Signal Builder : Subsystem  Tag=STV Subsys  Commented=on  LoadFcn=sigbuilder_block('load');  StartFcn=sigbuilder_block('start');  StopFcn=sigbuilder_block('stop');  ClipboardFcn=sigbuilder_block('clipboard');  mask(Sigbuilder block){}
      mask help: Simulink:masks:SigbuilderBlock_MD
      mask init:
      | if ~strcmp(get_param(bdroot(gcbh),'SimulationStatus'),'stopped') tuvar = sigbuilder_block('maskInit'); end
      settings: CopyFcn=sigbuilder_block('copy');  DeleteFcn=sigbuilder_block('delete');  ModelCloseFcn=sigbuilder_block('modelClose');  PreSaveFcn=sigbuilder_block('preSave');  PauseFcn=sigbuilder_block('pause');  ContinueFcn=sigbuilder_block('continue');  NameChangeFcn=sigbuilder_block('namechange');  OpenFcn=sigbuilder_block('open',[5.4 5.4 1141.2 580.8 ]);  CloseFcn=sigbuilder_block('close');
      mask Display: plot(0, 0, 100, 100,[2, 2, 32, 32, 2], [68, 8, 8, 68, 68],[32, 2], [38, 38], [32, 19, 2],[53, 60, 44], [32, 17, 17, 2],[16, 16, 31, 31]);txt = getActiveGroup(gcbh);text(2, 100, txt,'verticalAlignment', 'top');
  Subsystem : Subsystem
  Unary Minus1 : UnaryMinus
  Unit Delay : UnitDelay  InitialCondition=initial_pack_voltage  SampleTime=pack_voltage_sampling
  Unit Delay1 : UnitDelay  InitialCondition=initial_vehicle_side_voltage  SampleTime=vehicle_side_voltage_sampling
  Unit Delay2 : UnitDelay  InitialCondition=initial_pack_current  SampleTime=pack_current_sampling
  Unit Delay3 : UnitDelay  InitialCondition=initial_pack_soc  SampleTime=pack_soc_sampling
  Unit Delay4 : UnitDelay  InitialCondition=initial_cell_socs  SampleTime=cell_socs_sampling
  Unit Delay5 : UnitDelay  InitialCondition=initial_cell_ocvs  SampleTime=cell_ocvs_sampling
  Unit Delay6 : UnitDelay  InitialCondition=inital_outlet_temperature  SampleTime=pack_voltage_sampling
  Unit Delay8 : UnitDelay  InitialCondition=initial_cell_voltages  SampleTime=cell_voltages_sampling
  Unit Delay9 : UnitDelay  InitialCondition=initial_cell_temps  SampleTime=cell_temps_sampling
  cell_voltages : Outport
  cell_temperatures : Outport  Port=2
  cell_socs : Outport  Port=3
  cell_ocvs : Outport  Port=4
  pack_voltage : Outport  Port=5
  vehicle_side_voltage : Outport  Port=6
  pack_current : Outport  Port=7
  pack_soc : Outport  Port=8
  outlet_temperature : Outport  Port=9
  wires:
  Unit Delay/1 -> pack_voltage/1
  Unit Delay1/1 -> vehicle_side_voltage/1
  Unit Delay2/1 -> pack_current/1
  Unit Delay3/1 -> pack_soc/1
  Unit Delay8/1 -> cell_voltages/1
  Mux4/1 -> Unit Delay8/1
  Mux5/1 -> Unit Delay9/1
  Unit Delay9/1 -> cell_temperatures/1
  Mux1/1 -> Unit Delay4/1
  Unit Delay4/1 -> cell_socs/1
  Mux6/1 -> Unit Delay5/1
  Unit Delay5/1 -> cell_ocvs/1
  BatteryModelAdvanced/41(Cell_temp1) -> Mux5/1
  BatteryModelAdvanced/42(Cell_temp2) -> Mux5/2
  BatteryModelAdvanced/43(Cell_temp3) -> Mux5/3
  BatteryModelAdvanced/44(Cell_temp4) -> Mux5/4
  BatteryModelAdvanced/45(Cell_temp5) -> Mux5/5
  BatteryModelAdvanced/46(Cell_temp6) -> Mux5/6
  BatteryModelAdvanced/47(Cell_temp7) -> Mux5/7
  BatteryModelAdvanced/48(Cell_temp8) -> Mux5/8
  BatteryModelAdvanced/49(Cell_temp9) -> Mux5/9
  BatteryModelAdvanced/50(Cell_temp10) -> Mux5/10
  BatteryModelAdvanced/51(Cell_temp11) -> Mux5/11
  BatteryModelAdvanced/52(Cell_temp12) -> Mux5/12
  BatteryModelAdvanced/53(Cell_temp13) -> Mux5/13
  BatteryModelAdvanced/54(Cell_temp14) -> Mux5/14
  BatteryModelAdvanced/55(Cell_temp15) -> Mux5/15
  BatteryModelAdvanced/56(Cell_temp16) -> Mux5/16
  BatteryModelAdvanced/57(Cell_temp17) -> Mux5/17
  BatteryModelAdvanced/58(Cell_temp18) -> Mux5/18
  BatteryModelAdvanced/59(Cell_temp19) -> Mux5/19
  BatteryModelAdvanced/60(Cell_temp20) -> Mux5/20
  BatteryModelAdvanced/61(Cell_temp21) -> Mux5/21
  BatteryModelAdvanced/62(Cell_temp22) -> Mux5/22
  BatteryModelAdvanced/63(Cell_temp23) -> Mux5/23
  BatteryModelAdvanced/64(Cell_temp24) -> Mux5/24
  BatteryModelAdvanced/65(Cell_temp25) -> Mux5/25
  BatteryModelAdvanced/66(Cell_temp26) -> Mux5/26
  BatteryModelAdvanced/67(Cell_temp27) -> Mux5/27
  BatteryModelAdvanced/68(Cell_temp28) -> Mux5/28
  BatteryModelAdvanced/69(Cell_temp29) -> Mux5/29
  BatteryModelAdvanced/70(Cell_temp30) -> Mux5/30
  BatteryModelAdvanced/71(Cell_temp31) -> Mux5/31
  BatteryModelAdvanced/72(Cell_temp32) -> Mux5/32
  BatteryModelAdvanced/73(Cell_temp33) -> Mux5/33
  BatteryModelAdvanced/74(Cell_temp34) -> Mux5/34
  BatteryModelAdvanced/75(Cell_temp35) -> Mux5/35
  BatteryModelAdvanced/76(Cell_temp36) -> Mux5/36
  BatteryModelAdvanced/77(Cell_temp37) -> Mux5/37
  BatteryModelAdvanced/78(Cell_temp38) -> Mux5/38
  BatteryModelAdvanced/79(Cell_temp39) -> Mux5/39
  BatteryModelAdvanced/80(Cell_temp40) -> Mux5/40
  BatteryModelAdvanced/1(Cell_Voltage1) -> Mux4/1
  BatteryModelAdvanced/2(Cell_Voltage2) -> Mux4/2
  BatteryModelAdvanced/3(Cell_Voltage3) -> Mux4/3
  BatteryModelAdvanced/4(Cell_Voltage4) -> Mux4/4
  BatteryModelAdvanced/5(Cell_Voltage5) -> Mux4/5
  BatteryModelAdvanced/6(Cell_Voltage6) -> Mux4/6
  BatteryModelAdvanced/7(Cell_Voltage7) -> Mux4/7
  BatteryModelAdvanced/8(Cell_Voltage8) -> Mux4/8
  BatteryModelAdvanced/9(Cell_Voltage9) -> Mux4/9
  BatteryModelAdvanced/10(Cell_Voltage10) -> Mux4/10
  BatteryModelAdvanced/11(Cell_Voltage11) -> Mux4/11
  BatteryModelAdvanced/12(Cell_Voltage12) -> Mux4/12
  BatteryModelAdvanced/13(Cell_Voltage13) -> Mux4/13
  BatteryModelAdvanced/14(Cell_Voltage14) -> Mux4/14
  BatteryModelAdvanced/15(Cell_Voltage15) -> Mux4/15
  BatteryModelAdvanced/16(Cell_Voltage16) -> Mux4/16
  BatteryModelAdvanced/17(Cell_Voltage17) -> Mux4/17
  BatteryModelAdvanced/18(Cell_Voltage18) -> Mux4/18
  BatteryModelAdvanced/19(Cell_Voltage19) -> Mux4/19
  BatteryModelAdvanced/20(Cell_Voltage20) -> Mux4/20
  BatteryModelAdvanced/21(Cell_Voltage21) -> Mux4/21
  BatteryModelAdvanced/22(Cell_Voltage22) -> Mux4/22
  BatteryModelAdvanced/23(Cell_Voltage23) -> Mux4/23
  BatteryModelAdvanced/24(Cell_Voltage24) -> Mux4/24
  BatteryModelAdvanced/25(Cell_Voltage25) -> Mux4/25
  BatteryModelAdvanced/26(Cell_Voltage26) -> Mux4/26
  BatteryModelAdvanced/27(Cell_Voltage27) -> Mux4/27
  BatteryModelAdvanced/28(Cell_Voltage28) -> Mux4/28
  BatteryModelAdvanced/29(Cell_Voltage29) -> Mux4/29
  BatteryModelAdvanced/30(Cell_Voltage30) -> Mux4/30
  BatteryModelAdvanced/31(Cell_Voltage31) -> Mux4/31
  BatteryModelAdvanced/32(Cell_Voltage32) -> Mux4/32
  BatteryModelAdvanced/33(Cell_Voltage33) -> Mux4/33
  BatteryModelAdvanced/34(Cell_Voltage34) -> Mux4/34
  BatteryModelAdvanced/35(Cell_Voltage35) -> Mux4/35
  BatteryModelAdvanced/36(Cell_Voltage36) -> Mux4/36
  BatteryModelAdvanced/37(Cell_Voltage37) -> Mux4/37
  BatteryModelAdvanced/38(Cell_Voltage38) -> Mux4/38
  BatteryModelAdvanced/39(Cell_Voltage39) -> Mux4/39
  BatteryModelAdvanced/40(Cell_Voltage40) -> Mux4/40
  BatteryModelAdvanced/81(Cell_soc1) -> Mux1/1
  BatteryModelAdvanced/82(Cell_soc2) -> Mux1/2
  BatteryModelAdvanced/83(Cell_soc3) -> Mux1/3
  BatteryModelAdvanced/84(Cell_soc4) -> Mux1/4
  BatteryModelAdvanced/85(Cell_soc5) -> Mux1/5
  BatteryModelAdvanced/86(Cell_soc6) -> Mux1/6
  BatteryModelAdvanced/87(Cell_soc7) -> Mux1/7
  BatteryModelAdvanced/88(Cell_soc8) -> Mux1/8
  BatteryModelAdvanced/89(Cell_soc9) -> Mux1/9
  BatteryModelAdvanced/90(Cell_soc10) -> Mux1/10
  BatteryModelAdvanced/91(Cell_soc11) -> Mux1/11
  BatteryModelAdvanced/92(Cell_soc12) -> Mux1/12
  BatteryModelAdvanced/93(Cell_soc13) -> Mux1/13
  BatteryModelAdvanced/94(Cell_soc14) -> Mux1/14
  BatteryModelAdvanced/95(Cell_soc15) -> Mux1/15
  BatteryModelAdvanced/96(Cell_soc16) -> Mux1/16
  BatteryModelAdvanced/97(Cell_soc17) -> Mux1/17
  BatteryModelAdvanced/98(Cell_soc18) -> Mux1/18
  BatteryModelAdvanced/99(Cell_soc19) -> Mux1/19
  BatteryModelAdvanced/100(Cell_soc20) -> Mux1/20
  BatteryModelAdvanced/101(Cell_soc21) -> Mux1/21
  BatteryModelAdvanced/102(Cell_soc22) -> Mux1/22
  BatteryModelAdvanced/103(Cell_soc23) -> Mux1/23
  BatteryModelAdvanced/104(Cell_soc24) -> Mux1/24
  BatteryModelAdvanced/105(Cell_soc25) -> Mux1/25
  BatteryModelAdvanced/106(Cell_soc26) -> Mux1/26
  BatteryModelAdvanced/107(Cell_soc27) -> Mux1/27
  BatteryModelAdvanced/108(Cell_soc28) -> Mux1/28
  BatteryModelAdvanced/109(Cell_soc29) -> Mux1/29
  BatteryModelAdvanced/110(Cell_soc30) -> Mux1/30
  BatteryModelAdvanced/111(Cell_soc31) -> Mux1/31
  BatteryModelAdvanced/112(Cell_soc32) -> Mux1/32
  BatteryModelAdvanced/113(Cell_soc33) -> Mux1/33
  BatteryModelAdvanced/114(Cell_soc34) -> Mux1/34
  BatteryModelAdvanced/115(Cell_soc35) -> Mux1/35
  BatteryModelAdvanced/116(Cell_soc36) -> Mux1/36
  BatteryModelAdvanced/117(Cell_soc37) -> Mux1/37
  BatteryModelAdvanced/118(Cell_soc38) -> Mux1/38
  BatteryModelAdvanced/119(Cell_soc39) -> Mux1/39
  BatteryModelAdvanced/120(Cell_soc40) -> Mux1/40
  BatteryModelAdvanced/121(Cell_ocv1) -> Mux6/1
  BatteryModelAdvanced/122(Cell_ocv2) -> Mux6/2
  BatteryModelAdvanced/123(Cell_ocv3) -> Mux6/3
  BatteryModelAdvanced/124(Cell_ocv4) -> Mux6/4
  BatteryModelAdvanced/125(Cell_ocv5) -> Mux6/5
  BatteryModelAdvanced/126(Cell_ocv6) -> Mux6/6
  BatteryModelAdvanced/127(Cell_ocv7) -> Mux6/7
  BatteryModelAdvanced/128(Cell_ocv8) -> Mux6/8
  BatteryModelAdvanced/129(Cell_ocv9) -> Mux6/9
  BatteryModelAdvanced/130(Cell_ocv10) -> Mux6/10
  BatteryModelAdvanced/131(Cell_ocv11) -> Mux6/11
  BatteryModelAdvanced/132(Cell_ocv12) -> Mux6/12
  BatteryModelAdvanced/133(Cell_ocv13) -> Mux6/13
  BatteryModelAdvanced/134(Cell_ocv14) -> Mux6/14
  BatteryModelAdvanced/135(Cell_ocv15) -> Mux6/15
  BatteryModelAdvanced/136(Cell_ocv16) -> Mux6/16
  BatteryModelAdvanced/137(Cell_ocv17) -> Mux6/17
  BatteryModelAdvanced/138(Cell_ocv18) -> Mux6/18
  BatteryModelAdvanced/139(Cell_ocv19) -> Mux6/19
  BatteryModelAdvanced/140(Cell_ocv20) -> Mux6/20
  BatteryModelAdvanced/141(Cell_ocv21) -> Mux6/21
  BatteryModelAdvanced/142(Cell_ocv22) -> Mux6/22
  BatteryModelAdvanced/143(Cell_ocv23) -> Mux6/23
  BatteryModelAdvanced/144(Cell_ocv24) -> Mux6/24
  BatteryModelAdvanced/145(Cell_ocv25) -> Mux6/25
  BatteryModelAdvanced/146(Cell_ocv26) -> Mux6/26
  BatteryModelAdvanced/147(Cell_ocv27) -> Mux6/27
  BatteryModelAdvanced/148(Cell_ocv28) -> Mux6/28
  BatteryModelAdvanced/149(Cell_ocv29) -> Mux6/29
  BatteryModelAdvanced/150(Cell_ocv30) -> Mux6/30
  BatteryModelAdvanced/151(Cell_ocv31) -> Mux6/31
  BatteryModelAdvanced/152(Cell_ocv32) -> Mux6/32
  BatteryModelAdvanced/153(Cell_ocv33) -> Mux6/33
  BatteryModelAdvanced/154(Cell_ocv34) -> Mux6/34
  BatteryModelAdvanced/155(Cell_ocv35) -> Mux6/35
  BatteryModelAdvanced/156(Cell_ocv36) -> Mux6/36
  BatteryModelAdvanced/157(Cell_ocv37) -> Mux6/37
  BatteryModelAdvanced/158(Cell_ocv38) -> Mux6/38
  BatteryModelAdvanced/159(Cell_ocv39) -> Mux6/39
  BatteryModelAdvanced/160(Cell_ocv40) -> Mux6/40
  BatteryModelAdvanced/165(pack_soc) -> Unit Delay3/1
  BatteryModelAdvanced/164(pack_current) -> Unit Delay2/1
  BatteryModelAdvanced/163(vehicle_side_voltage) -> Unit Delay1/1
  BatteryModelAdvanced/162(pack_voltage) -> Unit Delay/1
  BatteryModelAdvanced/161(outlet_temperature) -> Unit Delay6/1
  Unit Delay6/1 -> outlet_temperature/1
  CB_cmds/1 -> Data Type Conversion6/1
  Data Type Conversion6/1 -> Demux/1
  Demux/1 -> BatteryModelAdvanced/1(cmd_1)
  Demux/2 -> BatteryModelAdvanced/2(cmd_2)
  Demux/3 -> BatteryModelAdvanced/3(cmd_3)
  Demux/4 -> BatteryModelAdvanced/4(cmd_4)
  Demux/5 -> BatteryModelAdvanced/5(cmd_5)
  Demux/6 -> BatteryModelAdvanced/6(cmd_6)
  Demux/7 -> BatteryModelAdvanced/7(cmd_7)
  Demux/8 -> BatteryModelAdvanced/8(cmd_8)
  Demux/9 -> BatteryModelAdvanced/9(cmd_9)
  Demux/10 -> BatteryModelAdvanced/10(cmd_10)
  Demux/11 -> BatteryModelAdvanced/11(cmd_11)
  Demux/12 -> BatteryModelAdvanced/12(cmd_12)
  Demux/13 -> BatteryModelAdvanced/13(cmd_13)
  Demux/14 -> BatteryModelAdvanced/14(cmd_14)
  Demux/15 -> BatteryModelAdvanced/15(cmd_15)
  Demux/16 -> BatteryModelAdvanced/16(cmd_16)
  Demux/17 -> BatteryModelAdvanced/17(cmd_17)
  Demux/18 -> BatteryModelAdvanced/18(cmd_18)
  Demux/19 -> BatteryModelAdvanced/19(cmd_19)
  Demux/20 -> BatteryModelAdvanced/20(cmd_20)
  Demux/21 -> BatteryModelAdvanced/21(cmd_21)
  Demux/22 -> BatteryModelAdvanced/22(cmd_22)
  Demux/23 -> BatteryModelAdvanced/23(cmd_23)
  Demux/24 -> BatteryModelAdvanced/24(cmd_24)
  Demux/25 -> BatteryModelAdvanced/25(cmd_25)
  Demux/26 -> BatteryModelAdvanced/26(cmd_26)
  Demux/27 -> BatteryModelAdvanced/27(cmd_27)
  Demux/28 -> BatteryModelAdvanced/28(cmd_28)
  Demux/29 -> BatteryModelAdvanced/29(cmd_29)
  Demux/30 -> BatteryModelAdvanced/30(cmd_30)
  Demux/31 -> BatteryModelAdvanced/31(cmd_31)
  Demux/32 -> BatteryModelAdvanced/32(cmd_32)
  Demux/33 -> BatteryModelAdvanced/33(cmd_33)
  Demux/34 -> BatteryModelAdvanced/34(cmd_34)
  Demux/35 -> BatteryModelAdvanced/35(cmd_35)
  Demux/36 -> BatteryModelAdvanced/36(cmd_36)
  Demux/37 -> BatteryModelAdvanced/37(cmd_37)
  Demux/38 -> BatteryModelAdvanced/38(cmd_38)
  Demux/39 -> BatteryModelAdvanced/39(cmd_39)
  Demux/40 -> BatteryModelAdvanced/40(cmd_40)
  pre_cc_cmd/1 -> Data Type Conversion1/1
  neg_cc_cmd/1 -> Data Type Conversion2/1
  chg_cc_cmd/1 -> Logical Operator/2, Data Type Conversion3/1
  fan_cmd/1 -> Data Type Conversion4/1
  cabin_temperature/1 -> Data Type Conversion5/1
  Data Type Conversion/1 -> BatteryModelAdvanced/41(main_cc_comd)
  Data Type Conversion1/1 -> BatteryModelAdvanced/42(pre_cc_cmd)
  Data Type Conversion2/1 -> BatteryModelAdvanced/43(neg_cc_cmd)
  Data Type Conversion3/1 -> BatteryModelAdvanced/44(chg_cc_cmd)
  Data Type Conversion4/1 -> BatteryModelAdvanced/45(fan_cmd)
  Data Type Conversion5/1 -> BatteryModelAdvanced/46(cabin_temp)
  Idischg_max/1 -> Unary Minus1/1
  Subsystem/1(input_I) -> Data Type Conversion9/1
  Data Type Conversion7/1 -> BatteryModelAdvanced/47(Ichg_max)
  Data Type Conversion8/1 -> BatteryModelAdvanced/48(Idischg_max)
  Data Type Conversion9/1 -> BatteryModelAdvanced/49(input_current)
  Data Type Conversion10/1 -> BatteryModelAdvanced/50(load_type)
  Unary Minus1/1 -> Data Type Conversion8/1
  main_cc_cmd/1 -> Logical Operator/1
  Logical Operator/1 -> Data Type Conversion/1
  Ichg_max/1 -> Data Type Conversion7/1, Subsystem/1(Ichg_max)
  From Workspace/1 -> Data Type Conversion10/1
